simulink model "main"  (R2016b)
settings: Solver=FixedStepAuto  StartTime=0.0  StopTime=inf  FixedStep=1e-3  RelTol=1e-3
values from neighbouring files (symbols this model uses):
  lx = 15    [platform_and_ball_characteristics.m]
  ly = 10    [platform_and_ball_characteristics.m]
libraries: MBDynCom x2, simulink x2
settings Model: Creator=matteo  LastModifiedBy=matteo

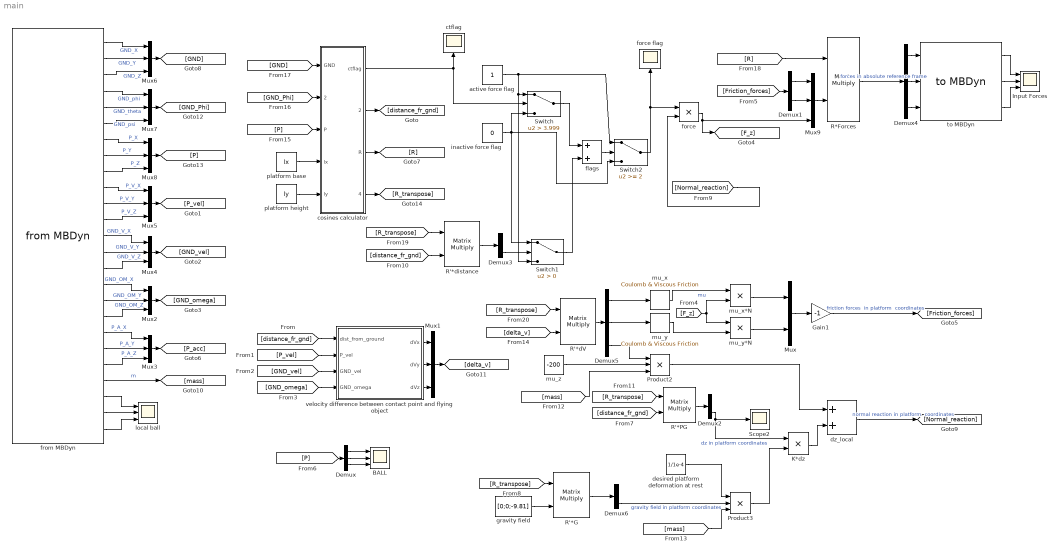
== system main ==
  BALL : Scope  NumInputPorts=3
  Demux{,2..6} (6 alike) : Demux  Outputs=3
  Demux1 : Demux  Outputs=2
  Gain1 : Gain  Gain=-1
  Input Forces : Scope  NumInputPorts=3
  K*dz : Product
  Mux : Mux  Inputs=2
  Mux{1..9} (9 alike) : Mux  Inputs=3
  Product2 : Product  Inputs=3
  Product3 : Product  Inputs=3
  R'*G : Product  Multiplication=Matrix(*)
  R'*PG : Product  Multiplication=Matrix(*)
  R'*dV : Product  Multiplication=Matrix(*)
  R'*distance : Product  Multiplication=Matrix(*)
  R*Forces : Product  Multiplication=Matrix(*)
  Scope2 : Scope
  Switch : Switch  Criteria=u2 > Threshold  Threshold=3.999
  Switch1 : Switch  Criteria=u2 > Threshold
  Switch2 : Switch  Threshold=2
  active force flag : Constant
  cosines calculator : MATLAB Function  TreatAsAtomicUnit=on
  ctflag : Scope
  desired platform deformation at rest : Constant  Value=1/1e-4
  dz_local : Sum
  flags : Sum
  force : Product
  force flag : Scope
  from MBDyn : MBDynCom/from MBDyn  Priority=0  RTAI_flag=off  Socket_flag=on  mbdtask='MBDTSK'  mbx='MBXINN'  net=on  node='127.0.0.1'  port=8000  path=''  N_chan=25  Tc=1.e-3
  gravity field : Constant  Value=[0;0;-9.81]
  inactive force flag : Constant  Value=0
  local ball : Scope  NumInputPorts=3
  mu_x : simulink/Discontinuities/Coulomb & Viscous Friction  offset=0  gain=0.05
  mu_x*N : Product
  mu_y : simulink/Discontinuities/Coulomb & Viscous Friction  offset=0  gain=0.05
  mu_y*N : Product
  mu_z : Constant  Value=-200
  platform base : Constant  Value=lx
  platform height : Constant  Value=ly
  to MBDyn : MBDynCom/to MBDyn  Priority=0  RTAI_flag=off  Socket_flag=on  mbdtask='MBDTSK'  mbx='MBXOUT'  net=on  node='127.0.0.1'  port=9000  path=''  N_chan=3  Tc=1e-3
  velocity difference between contact point and flying object : MATLAB Function  TreatAsAtomicUnit=on
  wires:
  to MBDyn/1 -> Input Forces/1
  from MBDyn/1 -> Mux6/1  "GND_X"
  from MBDyn/2 -> Mux6/2  "GND_Y"
  force/1 -> Mux9/3, [F_z]
  Switch/1 -> flags/1
  inactive force flag/1 -> Switch2/3, Switch1/1, Switch/3
  active force flag/1 -> Switch2/1, Switch1/3, Switch/1
  from MBDyn/10 -> Mux5/1  "P_V_X"
  from MBDyn/11 -> Mux5/2  "P_V_Y"
  from MBDyn/12 -> Mux5/3  "P_V_Z"
  from MBDyn/13 -> Mux4/1  "GND_V_X"
  from MBDyn/14 -> Mux4/2  "GND_V_Y"
  from MBDyn/15 -> Mux4/3  "GND_V_Z"
  from MBDyn/16 -> Mux2/1  "GND_OM_X"
  from MBDyn/17 -> Mux2/2  "GND_OM_Y"
  from MBDyn/18 -> Mux2/3  "GND_OM_Z"
  mu_x/1 -> mu_x*N/1  "mu"
  from MBDyn/19 -> Mux3/1  "P_A_X"
  from MBDyn/20 -> Mux3/2  "P_A_Y"
  from MBDyn/21 -> Mux3/3  "P_A_Z"
  from MBDyn/22 -> [mass]  "m"
  from MBDyn/4 -> Mux7/1  "GND_phi"
  from MBDyn/5 -> Mux7/2  "GND_theta"
  from MBDyn/6 -> Mux7/3  "GND_psi"
  [distance_fr_gnd] -> velocity difference between contact point and flying object/1(dist_from_ground)
  [P_vel] -> velocity difference between contact point and flying object/2(P_vel)
  [GND_vel] -> velocity difference between contact point and flying object/3(GND_vel)
  [GND_omega] -> velocity difference between contact point and flying object/4(GND_omega)
  Mux5/1 -> [P_vel]
  Mux4/1 -> [GND_vel]
  Mux2/1 -> [GND_omega]
  from MBDyn/3 -> Mux6/3  "GND_Z"
  from MBDyn/8 -> Mux8/2  "P_Y"
  from MBDyn/7 -> Mux8/1  "P_X"
  from MBDyn/9 -> Mux8/3  "P_Z"
  cosines calculator/2(distance_PG) -> [distance_fr_gnd]
  cosines calculator/1(ctflag) -> ctflag/1, Switch/2
  Demux/1 -> BALL/1
  Demux/2 -> BALL/2
  Demux/3 -> BALL/3
  [F_z] -> mu_x*N/2, mu_y*N/1
  mu_z/1 -> Product2/2
  [mass] -> Product2/3
  Demux1/1 -> Mux9/1
  Demux1/2 -> Mux9/2
  [Friction_forces] -> Demux1/1
  to MBDyn/2 -> Input Forces/2
  to MBDyn/3 -> Input Forces/3
  [P] -> Demux/1
  mu_y/1 -> mu_y*N/2
  mu_x*N/1 -> Mux/1
  mu_y*N/1 -> Mux/2
  Mux/1 -> Gain1/1
  [Normal_reaction] -> force/2
  cosines calculator/3(R) -> [R]
  [distance_fr_gnd] -> R'*PG/2
  Demux2/3 -> K*dz/1, Scope2/1  "dz in platform coordinates"
  Demux3/3 -> Switch1/2
  Switch2/1 -> force flag/1, force/1
  Switch1/1 -> flags/2
  flags/1 -> Switch2/2
  velocity difference between contact point and flying object/2(dVy) -> Mux1/2
  Mux1/1 -> [delta_v]
  velocity difference between contact point and flying object/1(dVx) -> Mux1/1
  velocity difference between contact point and flying object/3(dVz) -> Mux1/3
  Demux5/1 -> mu_x/1
  Demux5/2 -> mu_y/1
  Demux5/3 -> Product2/1
  Product2/1 -> dz_local/1
  dz_local/1 -> [Normal_reaction]  "normal reaction in platform  coordinates"
  [mass] -> Product3/3
  desired platform deformation at rest/1 -> Product3/1
  Product3/1 -> K*dz/2
  K*dz/1 -> dz_local/2
  Gain1/1 -> [Friction_forces]  "friction forces  in platform  coordinates"
  Mux8/1 -> [P]
  [P] -> cosines calculator/3(P)
  Mux7/1 -> [GND_Phi]
  [GND_Phi] -> cosines calculator/2(GND_Phi)
  [GND] -> cosines calculator/1(GND)
  Mux6/1 -> [GND]
  Mux3/1 -> [P_acc]
  from MBDyn/24 -> local ball/2
  from MBDyn/23 -> local ball/1
  from MBDyn/25 -> local ball/3
  R'*PG/1 -> Demux2/1
  [R_transpose] -> R'*PG/1
  cosines calculator/4(R_global_to_local) -> [R_transpose]
  [R_transpose] -> R'*G/1
  gravity field/1 -> R'*G/2
  R'*G/1 -> Demux6/1
  Mux9/1 -> R*Forces/2
  R*Forces/1 -> Demux4/1  "forces in absolute reference frame"
  Demux4/1 -> to MBDyn/1
  Demux4/2 -> to MBDyn/2
  Demux4/3 -> to MBDyn/3
  Demux6/3 -> Product3/2  "gravity field in platform coordinates"
  [distance_fr_gnd] -> R'*distance/2
  [R_transpose] -> R'*distance/1
  R'*distance/1 -> Demux3/1
  [R] -> R*Forces/1
  [R_transpose] -> R'*dV/1
  [delta_v] -> R'*dV/2
  R'*dV/1 -> Demux5/1
  platform height/1 -> cosines calculator/5(ly)
  platform base/1 -> cosines calculator/4(lx)

== matlab function main/velocity difference between contact point and flying object ==
  data: dist_from_ground input; dVx output; dVy output; P_vel input; GND_vel input; GND_omega input; dVz output
function [dVx,dVy,dVz] = fcn(dist_from_ground,P_vel,GND_vel,GND_omega)
%% MATTEO DANIELE
%  this function is intended to compute the relative velocity between the
%  contact point and the reference mass in order to model the surface
%  friction in a someway empirically

% distance between ground and "flying object" (for total speed)
% PG_distance = u(1:3);

% velocities useful to friction model
% P_vel = u(4:6);
% GND_vel = u(7:9);
% GND_omega = u(10:12);

% the contact point speed depends on the speed of GND node
V_Contact_Point = GND_vel + cross(GND_omega,dist_from_ground);

% speed difference between contact point and "flying object"
delta_V = P_vel-V_Contact_Point;

dVx = delta_V(1);
dVy = delta_V(2);
dVz = delta_V(3);

== matlab function main/cosines calculator ==
  data: GND input; ctflag output; GND_Phi input; P input; distance_PG output; lx input; ly input; R output; R_global_to_local output
function [ctflag,distance_PG,R,R_global_to_local] = fcn(GND,GND_Phi,P,lx,ly)
%% MATTEO DANIELE
% trying to create a contact constraint on platform that depends on the
% difference in position, speed, orientation and angular velocity between
% ground and "flying object"
n_vertices = 4;

% GND = [u(1);u(2);u(3)];
% GND_Phi = [u(4);u(5);u(6)];
% position of the point P ("flying object")
% P = [u(7);u(8);u(9)];

% rotation matrix to define all vertices
R = eul2rotm([GND_Phi(3) GND_Phi(2) GND_Phi(1)]);

% rotation matrix to define coordinates in the reference frame attached to
% the platfomr plane
R_global_to_local = R';
    
% initialization of z_normals and cosines
z_normals = zeros(3,n_vertices);
ct = zeros(1,n_vertices);
% initialization of distance vectors
PG = zeros(3,n_vertices);

% dimension of the platform along x 
% Length_x = u(10);
% dimension of the platform along y
% Length_y = u(11);

% rectangle of base Length_x and height Length_y
GND_vert = [ lx -lx -lx  lx
             ly  ly -ly -ly
              0  0   0   0  ];
               
for k = 1:n_vertices
    GND_vert(:,k) = GND + R*GND_vert(:,k);
%         distance vector between point and ground
        PG(:,k) = P-GND_vert(:,k);
%         normalization of the vector
        PG(:,k) = PG(:,k)/norm(PG(:,k));
end


% normals to planes
for k = 1:n_vertices-1
    z_normals(:,k) = cross(PG(:,k),PG(:,k+1));
    z_normals(:,k) = z_normals(:,k)/norm(z_normals(:,k));
end
z_normals(:,end) = cross(PG(:,end),PG(:,1));
z_normals(:,end) = z_normals(:,end)/norm(z_normals(:,end));

% platform plane normal (reference for cosine calculations)
z = cross(GND_vert(:,1)-GND,GND_vert(:,2)-GND);
z = z/norm(z);




% cosine of the angle between z and zij
for k = 1:n_vertices
    ct(k) = [z_normals(1,k) z_normals(2,k) z_normals(3,k)]*z;
end

% all cosines close to unit means that contact happens
ctflag = sum(ct);
% pass also the distance vector between "flying object" and ground
% reference point, it is useful to compute the arm for the angular speed of
% the velocity difference between point and platform
distance_PG = P-GND;

% ctflag close to 4 means that contact happens
% ideally when ctflag is 4 then contact happens, in reality ctflag must be
% over (or under) a certain limit to activate forces (eg: ctflag > 3.9)
% y(1,1) = ctflag;
% pass also the distance vector between "flying object" and ground
% reference point
% y(2:end,1) = P-GND;
